simulink subsystem "PVSystem"  (R2024a)
settings: Solver=VariableStepAuto  StartTime=0.0  StopTime=10  RelTol=1e-3
libraries: spsSeriesRLCBranchLib x2, spsBoostConverterLib x1, spsBreakerLib x1, simulink x1, spsCurrentMeasurementLib x1, spsGroundLib x1, spsPVArrayLib x1, spsVoltageMeasurementLib x1
settings Model: DefaultTestHarness=PVSystem_Harness1  Creator=nakamura  LastModifiedBy=nakamura

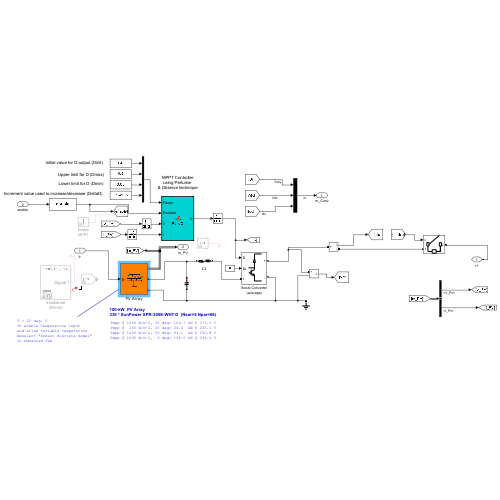
[thumbnail: Simulink's stored preview of the top-level diagram]
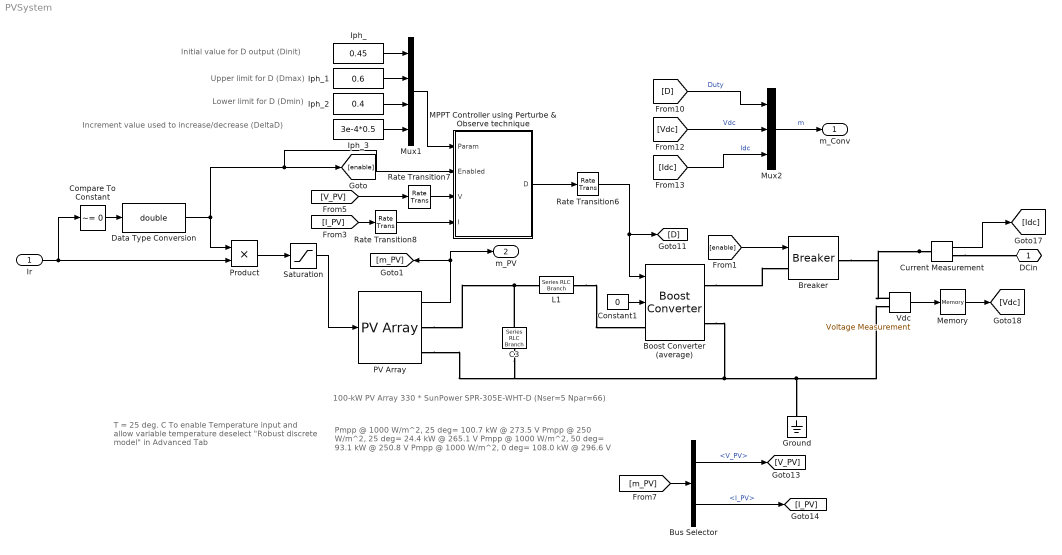
== system PVSystem ==
  note: Pmpp @ 1000 W/m^2, 25 deg= 100.7 kW @ 273.5 V
      | Pmpp @  250 W/m^2, 25 deg= 24.4  kW @ 265.1 V
      | Pmpp @ 1000 W/m^2, 50 deg= 93.1  kW @ 250.8 V
      | Pmpp @ 1000 W/m^2,  0 deg= 108.0 kW @ 296.6 V
  note: Lower limit for D (Dmin)
  note: 100-kW  PV Array
      | 330 * SunPower SPR-305E-WHT-D  (Nser=5 Npar=66)
  note: Increment value used to increase/decrease (DeltaD)
  note: Initial value for D output (Dinit)
  note: T = 25 deg. C
      | To enable Temperature input
      | and allow variable temperature
      | deselect "Robust discrete model"
      | in Advanced Tab
  note: Upper limit for D (Dmax)
  Ir : Inport
  Boost Converter (average) : spsBoostConverterLib/Boost Converter  ModelType=Average model (D-controlled)  Ron=1e-3  Rs=1e6  Cs=inf  Vforward=[0,0]  Ron_Diode=1e-7  Rs_Diode=1e7  Cs_Diode=inf  Vf_Diode=0  Rs_CurrentSource=inf  Ron_ACsource=1e-3
  Breaker : spsBreakerLib/Breaker  InitialState=0  SwitchingTimes="[1/60  5/60]"  External=on  BreakerResistance=1e-6  SnubberResistance=1e8  SnubberCapacitance=inf  Measurements=None  MoreParameters=on  NoBreakLoop=off
  Bus Selector : BusSelector  OutputSignals=V_PV,I_PV
  C3 : spsSeriesRLCBranchLib/Series RLC Branch  LConnTagsString=__new0  RConnTagsString=__new0  BranchType=C  Resistance=1.0  Inductance=1.0  SetiL0=off  InitialCurrent=0  Capacitance=100e-6  Setx0=off  InitialVoltage=0  Measurements=Branch voltage
  Compare To Constant : simulink/Logic and Bit Operations/Compare To Constant  relop=~=  const=0  OutDataTypeStr=boolean
  Constant1 : Constant  Value=0
  Current Measurement : spsCurrentMeasurementLib/Current Measurement  PhasorSimulation=off  OutputType=Complex  PSBequivalent=0
  Data Type Conversion : DataTypeConversion  OutDataTypeStr=double  SaturateOnIntegerOverflow=off  RndMeth=Floor
  Ground : spsGroundLib/Ground  LConnTagsString=a
  Iph_ : Constant  Value=0.45
  Iph_1 : Constant  Value=0.6
  Iph_2 : Constant  Value=0.4
  Iph_3 : Constant  Value=3e-4*0.5
  L1 : spsSeriesRLCBranchLib/Series RLC Branch  LConnTagsString=__new0  RConnTagsString=__new0  BranchType=RL  Resistance=0.005  Inductance=5e-3  SetiL0=off  InitialCurrent=0  Capacitance=1e-6  Setx0=off  InitialVoltage=0  Measurements=None
  "MPPT Controller using Perturbe & Observe technique " : MATLAB Function  TreatAsAtomicUnit=on
  Memory : Memory
  Mux1 : Mux
  Mux2 : Mux  Inputs=3
  PV Array : spsPVArrayLib/PV Array  Npar=66  Nser=5  PlotType=array @ 25 deg.C & specified irradiances  S_vec="[ 1000  250 ]"  Temp_C_vec=[ 0 25 50]  ModuleName=SunPower SPR-305E-WHT-D  PlotWhenSelected=off  Pm=305.226  Ncell=96  Voc=64.2  Isc=5.96  Vm=54.7  Im=5.58  beta_Voc_pc=-0.2727  alpha_Isc_pc=0.061745  beta_Voc=-0.17507  alpha_Isc=0.00368  IL=5.9657  I0=6.3076e-12  nI=0.94489  Rsh=393.2054  Rs=0.37428  RobustModel=on  RobustCellTemperature=25  BAL=off  Tc=10e-6  Tfilter=50e-6
  Product : Product
  Rate Transition6 : RateTransition  OutPortSampleTime=Ts_Power
  Rate Transition7 : RateTransition  OutPortSampleTime=Ts_Control
  Rate Transition8 : RateTransition  OutPortSampleTime=Ts_Control
  Saturation : Saturate  UpperLimit=inf  LowerLimit=0.1
  "Vdc " : spsVoltageMeasurementLib/Voltage Measurement  Tag=PoWeRsYsTeMmEaSuReMeNt  PhasorSimulation=off  OutputType=Magnitude  PSBequivalent=0
  DCin : PMIOPort  Side=Left
  m_Conv : Outport
  m_PV : Outport  Port=2
  wires:
  Iph_/1 -> Mux1/1
  Iph_2/1 -> Mux1/3
  Rate Transition8/1 -> "MPPT Controller using Perturbe & Observe technique "/4(I)
  PV Array/1 -> [m_PV], m_PV/1
  Constant1/1 -> Boost Converter (average)/2
  Mux1/1 -> "MPPT Controller using Perturbe & Observe technique "/1(Param)
  [I_PV] -> Rate Transition8/1
  [V_PV] -> Rate Transition7/1
  Rate Transition7/1 -> "MPPT Controller using Perturbe & Observe technique "/3(V)
  Iph_1/1 -> Mux1/2
  "MPPT Controller using Perturbe & Observe technique "/1(D) -> Rate Transition6/1
  Iph_3/1 -> Mux1/4
  Rate Transition6/1 -> [D], Boost Converter (average)/1
  Ir/1 -> Product/2, Compare To Constant/1
  [D] -> Mux2/1  "Duty"
  Mux2/1 -> m_Conv/1  "m"
  Current Measurement/1 -> [Idc]
  "Vdc "/1 -> Memory/1
  [Vdc] -> Mux2/2  "Vdc"
  [Idc] -> Mux2/3  "Idc"
  [m_PV] -> Bus Selector/1
  Bus Selector/1 -> [V_PV]  "<V_PV>"
  Bus Selector/2 -> [I_PV]  "<I_PV>"
  Data Type Conversion/1 -> Product/1, [enable], "MPPT Controller using Perturbe & Observe technique "/2(Enabled)
  Saturation/1 -> PV Array/1
  [enable] -> Breaker/1
  Compare To Constant/1 -> Data Type Conversion/1
  Product/1 -> Saturation/1
  Memory/1 -> [Vdc]
  connections:
  Boost Converter (average)/RConn2 -- PV Array/RConn2 -- C3/RConn1 -- "Vdc "/LConn2 -- Ground/LConn1
  C3/LConn1 -- L1/LConn1 -- PV Array/RConn1
  Current Measurement/LConn1 -- Breaker/RConn1 -- "Vdc "/LConn1
  L1/RConn1 -- Boost Converter (average)/LConn1
  Current Measurement/RConn1 -- DCin/RConn1
  Boost Converter (average)/RConn1 -- Breaker/LConn1

== matlab function PVSystem/MPPT Controller using Perturbe & Observe technique  ==
  settings: updateMethod=DISCRETE  sampleTime=Ts_Control
  data: Param input; Enabled input; V input; I input; D output
function D  = PandO(Param, Enabled, V, I)

% MPPT controller based on the Perturb & Observe algorithm.

% D output = Duty cycle of the boost converter (value between 0 and 1)
%
% Enabled input = 1 to enable the MPPT controller
% V input = PV array terminal voltage (V)
% I input = PV array current (A)
%
% Param input:
Dinit = Param(1);  %Initial value for D output
Dmax = Param(2);   %Maximum value for D
Dmin = Param(3);   %Minimum value for D
deltaD = Param(4); %Increment value used to increase/decrease the duty cycle D
% ( increasing D = decreasing Vref )
%  

persistent Vold Pold Dold;

dataType = 'double';

if isempty(Vold)
    Vold=0;
    Pold=0;
    Dold=Dinit;
end
P= V*I;
dV= V - Vold;
dP= P - Pold;

 if dP ~= 0 & Enabled ~=0
%     if dP>1e-9  & dP<-1e-9 & Enabled ~=0
    if dP < 0
        if dV < 0
            D = Dold - deltaD;
        else
            D = Dold + deltaD;
        end
    else
        if dV < 0
            D = Dold + deltaD;
        else
            D = Dold - deltaD;
        end    
    end
else D=Dold;
end

if D >= Dmax | D<= Dmin
    D=Dold;
end

Dold=D;
Vold=V;
Pold=P;
